simulink model "simulink_03"  (R2017b)
settings: Solver=ode45  StartTime=0.0  StopTime=30  RelTol=1e-3
undefined symbols (not defined in the file or in its folder): sigbuilder_block
settings Model: Creator=hp  LastModifiedBy=hp
settings DataIOCC: LimitDataPoints=on  SaveFormat=Array  Refine=10

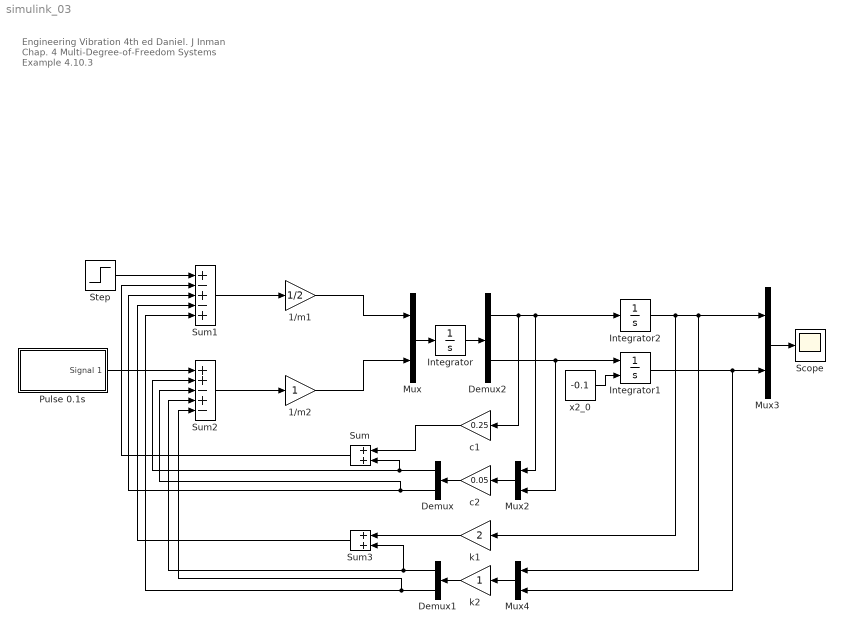
== system simulink_03 ==
  note: Engineering Vibration 4th ed Daniel. J Inman
      | Chap. 4 Multi-Degree-of-Freedom Systems
      | Example 4.10.3
  1/m1 : Gain  Gain=1/2
  1/m2 : Gain
  Demux : Demux  Outputs=2
  Demux1 : Demux  Outputs=2
  Demux2 : Demux  Outputs=2
  Integrator : Integrator
  Integrator1 : Integrator  InitialConditionSource=external  ContinuousStateAttributes='x2_0'
  Integrator2 : Integrator  ContinuousStateAttributes='x1_0'
  Mux{,2..4} (4 alike) : Mux  Inputs=2
  Pulse 0.1s : Subsystem  Tag=STV Subsys  LoadFcn=sigbuilder_block('load');  StartFcn=sigbuilder_block('start');  StopFcn=sigbuilder_block('stop');  ClipboardFcn=sigbuilder_block('clipboard');  mask(Sigbuilder block){tuvar=[0:10]}
      mask help: Simulink:masks:SigbuilderBlock_MD
      mask init:
      | if ~strcmp(get_param(bdroot(gcbh),'SimulationStatus'),'stopped') tuvar = sigbuilder_block('maskInit'); end
      settings: CopyFcn=sigbuilder_block('copy');  DeleteFcn=sigbuilder_block('delete');  ModelCloseFcn=sigbuilder_block('modelClose');  PreSaveFcn=sigbuilder_block('preSave');  PauseFcn=sigbuilder_block('pause');  ContinueFcn=sigbuilder_block('continue');  NameChangeFcn=sigbuilder_block('namechange');  OpenFcn=sigbuilder_block('open',[437.25 153 550.5 358.5 ]);  CloseFcn=sigbuilder_block('close');
      mask Display: plot(0, 0, 100, 100,[2, 2, 32, 32, 2], [68, 8, 8, 68, 68],[32, 2], [38, 38], [32, 19, 2],[53, 60, 44], [32, 17, 17, 2],[16, 16, 31, 31]);txt = getActiveGroup(gcbh);text(2, 100, txt,'verticalAlignment', 'top');
  Scope : Scope
  Step : Step  After=0  SampleTime=0
  Sum : Sum
  Sum1 : Sum  Inputs=+-+-+
  Sum2 : Sum  Inputs=++-+-
  Sum3 : Sum
  c1 : Gain  Gain=0.25
  c2 : Gain  Gain=0.05
  k1 : Gain  Gain=2
  k2 : Gain
  x2_0 : Constant  Value=-0.1
  wires:
  Step/1 -> Sum1/1
  Sum1/1 -> 1/m1/1
  Mux/1 -> Integrator/1
  Integrator/1 -> Demux2/1
  1/m1/1 -> Mux/1
  Demux2/1 -> c1/1, Mux2/1, Integrator2/1
  Demux2/2 -> Mux2/2, Integrator1/1
  1/m2/1 -> Mux/2
  Sum2/1 -> 1/m2/1
  Mux2/1 -> c2/1
  c1/1 -> Sum/1
  Sum/1 -> Sum1/2
  c2/1 -> Demux/1
  Demux/1 -> Sum2/2, Sum/2
  Demux/2 -> Sum2/3, Sum1/3
  Integrator2/1 -> k1/1, Mux4/1, Mux3/1
  Integrator1/1 -> Mux4/2, Mux3/2
  Mux3/1 -> Scope/1
  k1/1 -> Sum3/1
  Mux4/1 -> k2/1
  k2/1 -> Demux1/1
  Demux1/1 -> Sum3/2, Sum2/4
  Sum3/1 -> Sum1/4
  Demux1/2 -> Sum2/5, Sum1/5
  Pulse 0.1s/1(Signal 1) -> Sum2/1
  x2_0/1 -> Integrator1/2

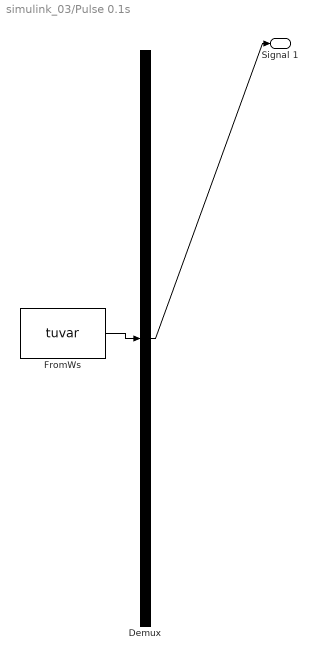
== system simulink_03/Pulse 0.1s ==
  Demux : Demux  Tag=STV Demux  Outputs=1
  FromWs : FromWorkspace  Tag=STV FromWs  VariableName=tuvar  SampleTime=0
      SigBuilderData=|
      | common.afterFinalStr = 'Extrapolate'
      | common.sampleTime = 0
      | dataSet.timeRange = [0 10]
      | dataSet.name = 'Group 1'
      | sbobj.Groups.Name = 'Group 1'
      | sbobj.Groups.Signals.Name = 'Signal 1'
      | sbobj.Groups.Signals.XData = [0 1 1 1.1 1.1 10]
      | sbobj.Groups.Signals.YData = [0 0 1 1 0 0]
  Signal 1 : Outport  Tag=STV Outport
  wires:
  FromWs/1 -> Demux/1
  Demux/1 -> Signal 1/1
